simulink model "ACCSoftwareComposition"  (R2024b)
settings: Solver=FixedStepDiscrete  StartTime=0.0  StopTime=10.0  RelTol=1e-3  EnableMultiTasking=on
settings Model: Creator=denis  LastModifiedBy=denis
settings OptimizationCC: DefaultParameterBehavior=Inlined  UseDivisionForNetSlopeComputation=on  GainParamInheritBuiltInType=on  UseFloatMulNetSlope=on  InlineInvariantSignals=on  PassReuseOutputArgsAs=Individual arguments  ZeroExternalMemoryAtStartup=off  ZeroInternalMemoryAtStartup=off  NoFixptDivByZeroProtection=on  EfficientFloat2IntCast=on  LifeSpan=1  OptimizeBlockOrder=speed  DifferentSizesBufferReuse=on  EfficientTunableParamExpr=on
settings DebuggingCC: ParameterTunabilityLossMsg=error
settings HardwareCC: ProdLongLongMode=on
settings SFSimCC: MATLABDynamicMemAlloc=off
settings RTWCC: Description=Embedded Coder  SystemTargetFile=ert.tlc  TemplateMakefile=ert_default_tmf  TargetLang=C++
settings CodeAppCC: ForceParamTrailComments=on  IgnoreCustomStorageClasses=off  OperatorAnnotations=on  SimulinkDataObjDesc=on  SFDataObjDesc=on  CustomSymbolStrGlobalVar=rt$N$M  CustomSymbolStrType=$N$M  CustomSymbolStrFcn=$N$M$F  CustomSymbolStrMacro=$N$M  InsertBlockDesc=on
settings ERTTargetCC: TargetLangStandard=C++11 (ISO)  GenerateSampleERTMain=on  IncludeMdlTerminateFcn=off  CombineSignalStateStructs=on  SuppressErrorStatus=on  SupportAbsoluteTime=off  CodeInterfacePackaging=C++ class  SupportComplex=off  RootIOFormat=Structure reference  ERTCustomFileTemplate=example_file_process.tlc  ERTFilePackagingFormat=CompactWithDataFile

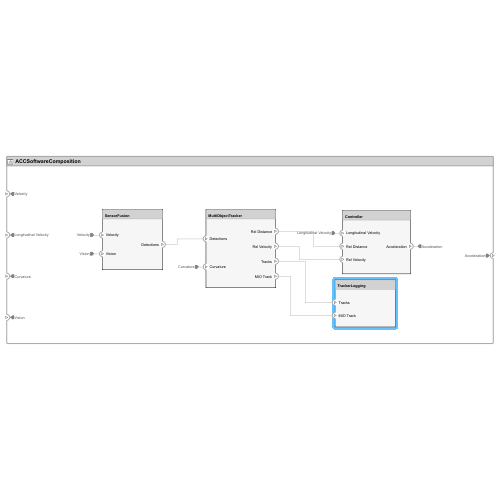
[thumbnail: Simulink's stored preview of the top-level diagram]
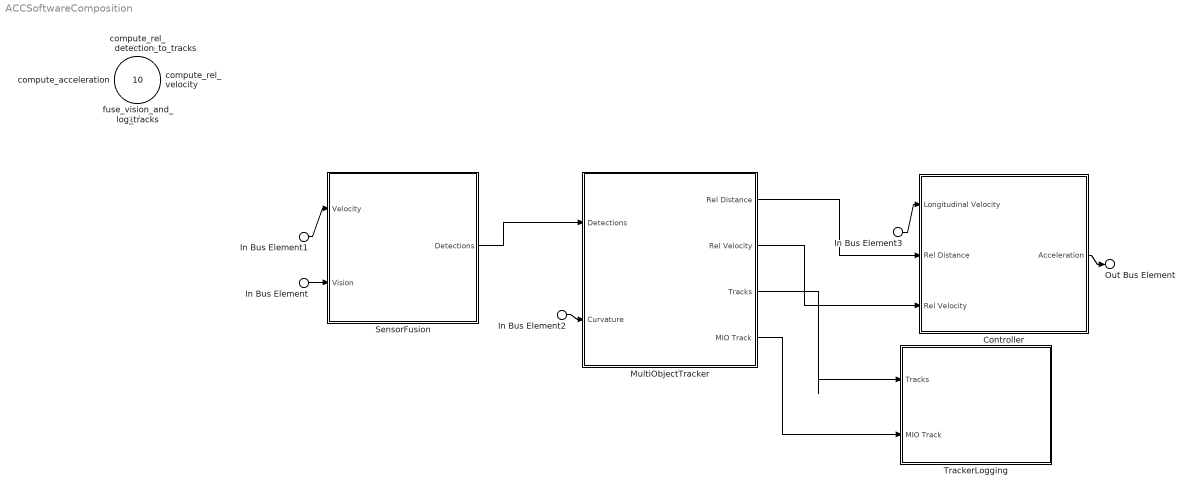
== system ACCSoftwareComposition ==
  In Bus Element1 : Inport  PortName=Velocity
  In Bus Element3 : Inport  Port=2  PortName=Longitudinal Velocity
  In Bus Element2 : Inport  Port=3  PortName=Curvature
  In Bus Element : Inport  Port=4  PortName=Vision
  fuse_vision_and_radar : Inport  Port=5  SampleTime=0.1  OutputFunctionCall=on
  compute_rel_distance : Inport  Port=6  SampleTime=0.1  OutputFunctionCall=on
  compute_rel_velocity : Inport  Port=7  SampleTime=0.1  OutputFunctionCall=on
  compute_acceleration : Inport  Port=8  SampleTime=0.1  OutputFunctionCall=on
  detection_to_tracks : Inport  Port=9  SampleTime=0.1  OutputFunctionCall=on
  log_tracks : Inport  Port=10  SampleTime=0.2  OutputFunctionCall=on
  Controller : Subsystem
      settings: PortSchema="{\"entries\":[{\"content\":{\"headerSize\":26,\"margin\":15,\"minimumSpacing\":25,\"sides\":[{\"content\":{\"connectorIds\":[\"In1\",\"In2\",\"In3\"]},\"type\":\"ConnectorPlacement.EquallySpacedRectSide\",\"uuid\":\"0d61c93e-5417-4b7d-8fa9-42b8d65d8ca8\"},{\"content\":{\"connectorIds\":[\"Out1\"],\"side\":\"RIGHT\"},\"type\":\"ConnectorPlacement.EquallySpacedRectSide\",\"uuid\":\"7aff60b2-8d48-4daa-8043-31aef3573339\"},{\"content\":{\"side\":\"TOP\"},\"type\":\"ConnectorPlacement.EquallySpacedRectSide\",\"uuid\":\"0a05ee61-d742-4f21-b4e7-616c02a34363\"}]},\"type\":\"ConnectorPlacement.EquallySpacedConnector\",\"uuid\":\"520a1049-b0db-4d40-9f8d-a6ea5b81fbfd\"}],\"packageUris\":[\"http://schema.mathworks.com/mf0/Connector/R2020b\"],\"version\":\"1.0\"}"
  MultiObjectTracker : Subsystem
      settings: PortSchema="{\"entries\":[{\"content\":{\"headerSize\":26,\"margin\":15,\"minimumSpacing\":25,\"sides\":[{\"content\":{\"connectorIds\":[\"In1\",\"In2\"]},\"type\":\"ConnectorPlacement.EquallySpacedRectSide\",\"uuid\":\"0d61c93e-5417-4b7d-8fa9-42b8d65d8ca8\"},{\"content\":{\"connectorIds\":[\"Out1\",\"Out2\",\"Out3\",\"Out4\"],\"side\":\"RIGHT\"},\"type\":\"ConnectorPlacement.EquallySpacedRectSide\",\"uuid\":\"7aff60b2-8d48-4daa-8043-31aef3573339\"},{\"content\":{\"side\":\"TOP\"},\"type\":\"ConnectorPlacement.EquallySpacedRectSide\",\"uuid\":\"0a05ee61-d742-4f21-b4e7-616c02a34363\"}]},\"type\":\"ConnectorPlacement.EquallySpacedConnector\",\"uuid\":\"520a1049-b0db-4d40-9f8d-a6ea5b81fbfd\"}],\"packageUris\":[\"http://schema.mathworks.com/mf0/Connector/R2020b\"],\"version\":\"1.0\"}"
  SensorFusion : Subsystem
      settings: PortSchema="{\"entries\":[{\"content\":{\"headerSize\":26,\"margin\":15,\"minimumSpacing\":25,\"sides\":[{\"content\":{\"connectorIds\":[\"In1\",\"In2\"]},\"type\":\"ConnectorPlacement.EquallySpacedRectSide\",\"uuid\":\"0d61c93e-5417-4b7d-8fa9-42b8d65d8ca8\"},{\"content\":{\"connectorIds\":[\"Out1\"],\"side\":\"RIGHT\"},\"type\":\"ConnectorPlacement.EquallySpacedRectSide\",\"uuid\":\"7aff60b2-8d48-4daa-8043-31aef3573339\"},{\"content\":{\"side\":\"TOP\"},\"type\":\"ConnectorPlacement.EquallySpacedRectSide\",\"uuid\":\"0a05ee61-d742-4f21-b4e7-616c02a34363\"}]},\"type\":\"ConnectorPlacement.EquallySpacedConnector\",\"uuid\":\"520a1049-b0db-4d40-9f8d-a6ea5b81fbfd\"}],\"packageUris\":[\"http://schema.mathworks.com/mf0/Connector/R2020b\"],\"version\":\"1.0\"}"
  TrackerLogging : Subsystem
      settings: PortSchema="{\"entries\":[{\"content\":{\"headerSize\":26,\"margin\":15,\"minimumSpacing\":25,\"sides\":[{\"content\":{\"connectorIds\":[\"In1\",\"In2\"]},\"type\":\"ConnectorPlacement.EquallySpacedRectSide\",\"uuid\":\"0d61c93e-5417-4b7d-8fa9-42b8d65d8ca8\"},{\"content\":{\"side\":\"RIGHT\"},\"type\":\"ConnectorPlacement.EquallySpacedRectSide\",\"uuid\":\"7aff60b2-8d48-4daa-8043-31aef3573339\"},{\"content\":{\"side\":\"TOP\"},\"type\":\"ConnectorPlacement.EquallySpacedRectSide\",\"uuid\":\"0a05ee61-d742-4f21-b4e7-616c02a34363\"}]},\"type\":\"ConnectorPlacement.EquallySpacedConnector\",\"uuid\":\"520a1049-b0db-4d40-9f8d-a6ea5b81fbfd\"}],\"packageUris\":[\"http://schema.mathworks.com/mf0/Connector/R2020b\"],\"version\":\"1.0\"}"
  Out Bus Element : Outport  PortName=Acceleration
  wires:
  In Bus Element/1 -> SensorFusion/2(Vision)
  In Bus Element1/1 -> SensorFusion/1(Velocity)
  SensorFusion/1(Detections) -> MultiObjectTracker/1(Detections)
  In Bus Element2/1 -> MultiObjectTracker/2(Curvature)
  MultiObjectTracker/1(Rel Distance) -> Controller/2(Rel Distance)
  MultiObjectTracker/2(Rel Velocity) -> Controller/3(Rel Velocity)
  MultiObjectTracker/4(MIO Track) -> TrackerLogging/2(MIO Track)
  MultiObjectTracker/3(Tracks) -> TrackerLogging/1(Tracks)
  In Bus Element3/1 -> Controller/1(Longitudinal Velocity)
  Controller/1(Acceleration) -> Out Bus Element/1

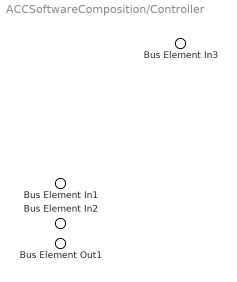
== system ACCSoftwareComposition/Controller ==
  Bus Element In3 : Inport  PortName=Longitudinal Velocity
  Bus Element In1 : Inport  Port=2  PortName=Rel Distance
  Bus Element In2 : Inport  Port=3  PortName=Rel Velocity
  Bus Element Out1 : Outport  PortName=Acceleration

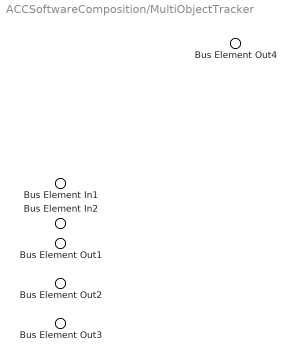
== system ACCSoftwareComposition/MultiObjectTracker ==
  Bus Element In1 : Inport  PortName=Detections
  Bus Element In2 : Inport  Port=2  PortName=Curvature
  Bus Element Out1 : Outport  PortName=Rel Distance
  Bus Element Out2 : Outport  Port=2  PortName=Rel Velocity
  Bus Element Out4 : Outport  Port=3  PortName=Tracks
  Bus Element Out3 : Outport  Port=4  PortName=MIO Track

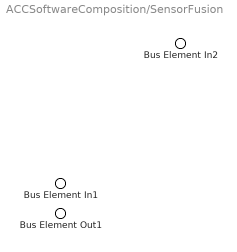
== system ACCSoftwareComposition/SensorFusion ==
  Bus Element In2 : Inport  PortName=Velocity
  Bus Element In1 : Inport  Port=2  PortName=Vision
  Bus Element Out1 : Outport  PortName=Detections

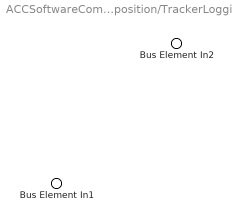
== system ACCSoftwareComposition/TrackerLogging ==
  Bus Element In2 : Inport  PortName=Tracks
  Bus Element In1 : Inport  Port=2  PortName=MIO Track
